simulink model "Sketch"  (R2022b)
settings: Solver=VariableStepAuto  StartTime=0.0  StopTime=10.0  RelTol=1e-3
PreLoadFcn:
  | run("Fzg_par.m")
settings Model: LastModifiedBy=timos
settings OptimizationCC: ReuseModelBlockBuffer=on
settings RTWCC: GPUComputeCapability=5.0
settings ConfigComp: CovBoundaryAbsTol=1.0e-5

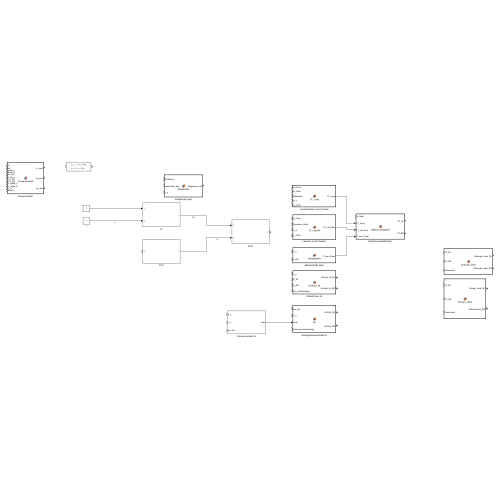
[thumbnail: Simulink's stored preview of the top-level diagram]
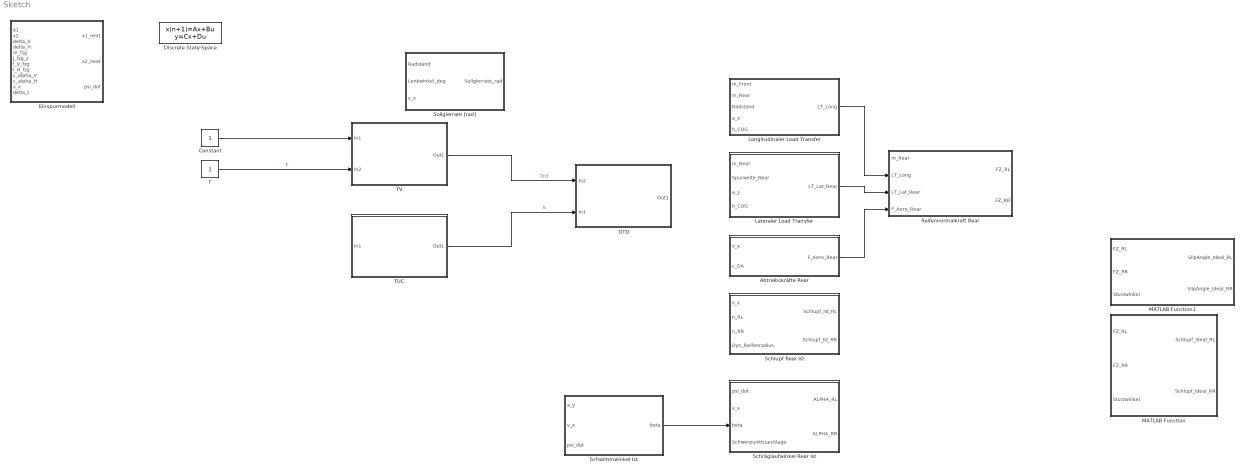
== system Sketch ==
  Abtriebskräfte Rear : MATLAB Function  TreatAsAtomicUnit=on
  Constant : Constant
  DTD : Subsystem
  Discrete State-Space : DiscreteStateSpace  SampleTime=-1
  Einspurmodell : MATLAB Function  TreatAsAtomicUnit=on
  Lateraler Load Transfer : MATLAB Function  TreatAsAtomicUnit=on
  Longitudinaler Load Transfer : MATLAB Function  TreatAsAtomicUnit=on
  MATLAB Function : MATLAB Function  TreatAsAtomicUnit=on
  MATLAB Function1 : MATLAB Function  TreatAsAtomicUnit=on
  Reifennormalkraft Rear : MATLAB Function  TreatAsAtomicUnit=on
  Schlupf Rear Ist : MATLAB Function  TreatAsAtomicUnit=on
  Schräglaufwinkel Rear Ist : MATLAB Function  TreatAsAtomicUnit=on
  Schwimmwinkel Ist : Subsystem
  Sollgierrate [rad] : MATLAB Function  TreatAsAtomicUnit=on
  TUC : Subsystem
  TV : Subsystem
  Γ : Constant
  wires:
  TUC/1(Out1) -> DTD/2(In1)  "S"
  TV/1(Out1) -> DTD/1(In2)  "Γr/l"
  Constant/1 -> TV/1(In1)
  Γ/1 -> TV/2(In2)  "Γ"
  Longitudinaler Load Transfer/1(LT_Long) -> Reifennormalkraft Rear/2(LT_Long)
  Lateraler Load Transfer/1(LT_Lat_Rear) -> Reifennormalkraft Rear/3(LT_Lat_Rear)
  Abtriebskräfte Rear/1(F_Aero_Rear) -> Reifennormalkraft Rear/4(F_Aero_Rear)
  Schwimmwinkel Ist/1(beta) -> Schräglaufwinkel Rear Ist/3(beta)

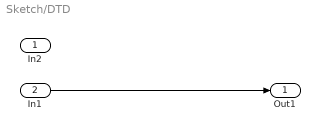
== system Sketch/DTD ==
  In2 : Inport
  In1 : Inport  Port=2
  Out1 : Outport
  wires:
  In1/1 -> Out1/1

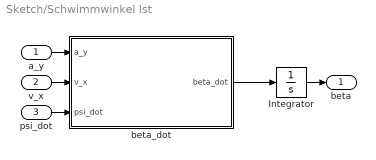
== system Sketch/Schwimmwinkel Ist ==
  a_y : Inport
  v_x : Inport  Port=2
  psi_dot : Inport  Port=3
  Integrator : Integrator
  beta_dot : MATLAB Function  TreatAsAtomicUnit=on
  beta : Outport
  wires:
  v_x/1 -> beta_dot/2(v_x)
  a_y/1 -> beta_dot/1(a_y)
  psi_dot/1 -> beta_dot/3(psi_dot)
  beta_dot/1(beta_dot) -> Integrator/1
  Integrator/1 -> beta/1

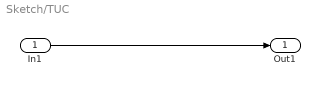
== system Sketch/TUC ==
  In1 : Inport
  Out1 : Outport
  wires:
  In1/1 -> Out1/1

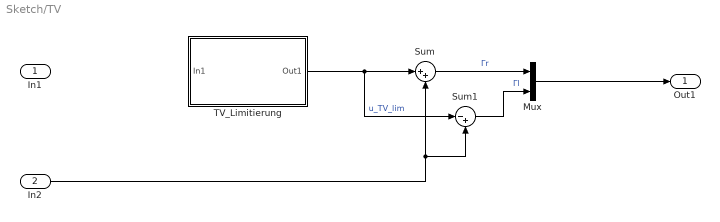
== system Sketch/TV ==
  In1 : Inport
  In2 : Inport  Port=2
  Mux : Mux  Inputs=2
  Sum : Sum  Inputs=|++
  Sum1 : Sum  Inputs=|-+
  TV_Limitierung : Subsystem
  Out1 : Outport
  wires:
  TV_Limitierung/1(Out1) -> Sum1/1, Sum/1  "u_TV_lim"
  In2/1 -> Sum1/2, Sum/2
  Sum/1 -> Mux/1  "Γr"
  Sum1/1 -> Mux/2  "Γl"
  Mux/1 -> Out1/1

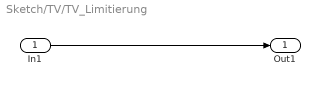
== system Sketch/TV/TV_Limitierung ==
  In1 : Inport
  Out1 : Outport
  wires:
  In1/1 -> Out1/1

== matlab function Sketch/Schräglaufwinkel Rear Ist ==
  data: psi_dot input; ALPHA_RL output; ALPHA_RR output; v_x input; beta input; Schwerpunktruecklage input
function [ALPHA_RL,ALPHA_RR] = fcn(psi_dot,v_x,beta,Schwerpunktruecklage)

    ALPHA_RL = (psi_dot*Schwerpunktruecklage/v_x) + beta;
    ALPHA_RR = ALPHA_RL;

== matlab function Sketch/Schwimmwinkel Ist/beta_dot ==
  data: a_y input; beta_dot output; v_x input; psi_dot input
function beta_dot  = Schwimmwinkel(a_y,v_x,psi_dot)

    beta_dot = (a_y/v_x) - psi_dot;

== matlab function Sketch/MATLAB Function1 ==
  data: FZ_RL input; SlipAngle_Ideal_RL output; FZ_RR input; Sturzwinkel input; SlipAngle_Ideal_RR output
function [SlipAngle_Ideal_RL,SlipAngle_Ideal_RR] = Schlupf_Ideal(FZ_RL,FZ_RR,Sturzwinkel)
% Scaling und Shape Koeffizienten
LCY   				= 0.90;
LMUY  				= 0.75;
LEY   				= 1;
LKY   				= 1;
LHY   				= 0;
LVY   				= 0;
LGAY  				= 0.75;
% Laterale Koeffizienten
PCY1				= +1.625E+000;
PDY1				= +2.554E+000;
PDY2				= -4.021E-001;
PDY3				= +5.406E+000;
PEY1				= +1.715E-001;
PEY2				= -8.339E-001;
PEY3				= -1.743E-001;
PEY4				= -6.110E+000;
PKY1				= -5.912E+001;
PKY2				= +2.567E+000;
PKY3				= +4.787E-001;
PHY1				= +0.000E+000;
PHY2				= +0.000E+000;
PHY3				= -2.152E-002;
PVY1				= +0.000E+000;
PVY2				= +0.000E+000;
PVY3				= -2.151E+000;
PVY4				= -8.772E-001;
% =======================================================================
% RL
i = 0;
Fz = FZ_RL;
GAMMA = Sturzwinkel;
FY_RL = zeros((12/0.1),3);                                                  % Vorinitialisierung
for ALPHA = 0:0.1:12
    % ====================================================================
    % Magic Formula Berechnung FX // Nur Längsschlupf
    GAMMAY = GAMMA .* LGAY;
    SHY = (PHY1 + PHY2 .* DFZ) .* LHY + PHY3 .* GAMMAY;
    ALPHAY = ALPHA + SHY;
    CY = PCY1 .* LCY;
    MUY = (PDY1 + PDY2 .* DFZ) .* (1 - PDY3 .* GAMMAY.^2) .* LMUY;
    DY = MUY .* Fz;
    EY = (PEY1 + PEY2 .* DFZ) .* (1 - (PEY3 + PEY4 .* GAMMAY) .* sign(ALPHAY)) .* LEY;
    KY = PKY1 .* FZ0 .* sin(2 * atan(Fz ./ (PKY2 .* FZ0 .* LFZO))) .* (1 - PKY3 .* abs(GAMMAY)) .* LFZO .* LKY;
    BY = KY ./ (CY .* DY);
    SVY = Fz .* ((PVY1 + PVY2 .* DFZ) .* LVY + (PVY3 + PVY4 .* DFZ) .* GAMMAY) .* LMUY;
    % ====================================================================
    % Eintragung in die Matrix
    i=i+1;
    FY_RL(i,1) = Fz;
    FY_RL(i,2) = ALPHA;
    FY_RL(i,3) = DY .* sin(CY .* atan(BY .* ALPHAY - EY .* (BY .* ALPHAY - atan(BY .* ALPHAY)))) + SVY;
end
[~, Index] = max(FY_RL(:,3));                                               % Zeilennummer des maximalen FX-Werte
SlipAngle_Ideal_RL = FY_RL(Index,2);                                        % Eintragung in die Ausgabegröße
% =======================================================================
% RR
i = 0;
Fz = FZ_RR;
GAMMA = Sturzwinkel;
FY_RR = zeros((12/0.1),3);                                                  % Vorinitialisierung
for ALPHA = 0:0.1:12
    % ====================================================================
    % Magic Formula Berechnung FX // Nur Längsschlupf
    GAMMAY = GAMMA .* LGAY;
    SHY = (PHY1 + PHY2 .* DFZ) .* LHY + PHY3 .* GAMMAY;
    ALPHAY = ALPHA + SHY;
    CY = PCY1 .* LCY;
    MUY = (PDY1 + PDY2 .* DFZ) .* (1 - PDY3 .* GAMMAY.^2) .* LMUY;
    DY = MUY .* Fz;
    EY = (PEY1 + PEY2 .* DFZ) .* (1 - (PEY3 + PEY4 .* GAMMAY) .* sign(ALPHAY)) .* LEY;
    KY = PKY1 .* FZ0 .* sin(2 * atan(Fz ./ (PKY2 .* FZ0 .* LFZO))) .* (1 - PKY3 .* abs(GAMMAY)) .* LFZO .* LKY;
    BY = KY ./ (CY .* DY);
    SVY = Fz .* ((PVY1 + PVY2 .* DFZ) .* LVY + (PVY3 + PVY4 .* DFZ) .* GAMMAY) .* LMUY;
    % ====================================================================
    % Eintragung in die Matrix
    i=i+1;
    FY_RR(i,1) = Fz;
    FY_RR(i,2) = ALPHA;
    FY_RR(i,3) = DY .* sin(CY .* atan(BY .* ALPHAY - EY .* (BY .* ALPHAY - atan(BY .* ALPHAY)))) + SVY;
end
[~, Index] = max(FY_RR(:,3));                                               % Zeilennummer des maximalen FX-Werte
SlipAngle_Ideal_RR = FY_RR(Index,2);                                        % Eintragung in die Ausgabegröße

== matlab function Sketch/MATLAB Function ==
  data: FZ_RL input; Schlupf_Ideal_RL output; FZ_RR input; Sturzwinkel input; Schlupf_Ideal_RR output
function [Schlupf_Ideal_RL,Schlupf_Ideal_RR] = Schlupf_Ideal(FZ_RL,FZ_RR,Sturzwinkel)
% =======================================================================
% Magic Formula Parameter
% Scaling und Shape Koeffizienten
LCX   				= 1;
LMUX  				= 0.75;
LEX   				= 1;
LKX   				= 1;
LHX   				= 1;
LVX   				= 1;
LGAX  				= 1;
% Longitudinal Koeffizienten
PCX1  				= +1.786E+000;
PDX1  				= +2.688E+000;
PDX2  				= -2.720E-001;
PDX3  				= +1.370E+001;
PEX1  				= +8.710E-001;
PEX2  				= -3.800E-002;
PEX3  				= +0.000E+000;
PEX4  				= +7.100E-002;
PKX1  				= +8.125E+001;
PKX2  				= -2.025E+001;
PKX3  				= +5.000E-001;
PHX1  				= +0.000E+000;
PHX2  				= +0.000E+000;
PVX1  				= +0.000E+000;
PVX2  				= +0.000E+000;
% =======================================================================
% RL
i = 0;
Fz = FZ_RL;
GAMMA = Sturzwinkel;
FX_RL = zeros((0.3/0.01),3);                                                % Vorinitialisierung
for KAPPA = 0:0.01:0.3
    % ====================================================================
    % Magic Formula Berechnung FX // Nur Längsschlupf
    GAMMAX = GAMMA .* LGAX;
    SHX = (PHX1 + PHX2 .* DFZ) .* LHX;
    KAPPAX = KAPPA + SHX;
    CX = PCX1 .* LCX;
    MUX = (PDX1 + PDX2 .* DFZ) .* (1 - PDX3 .* GAMMAX.^2) .* LMUX;
    DX = MUX .* Fz;
    EX = (PEX1 + PEX2 .* DFZ + PEX3 .* DFZ.^2) .* (1 - PEX4 .* sign(KAPPAX)) .* LEX;
    KX = Fz .* (PKX1 + PKX2 .* DFZ) .* exp(PKX3 .* DFZ) .* LKX;
    BX = KX ./ (CX .* DX);
    SVX = Fz .* (PVX1 + PVX2 .* DFZ) .* LVX .* LMUX;
    % ====================================================================
    % Eintragung in die Matrix
    i=i+1;
    FX_RL(i,1) = Fz;
    FX_RL(i,2) = KAPPA;
    FX_RL(i,3) = DX .* sin(CX .* atan(BX .* KAPPAX - EX .* (BX .* KAPPAX - atan(BX .* KAPPAX)))) + SVX;
end
[~, Index] = max(FX_RL(:,3));                                               % Zeilennummer des maximalen FX-Werte
Schlupf_Ideal_RL = FX_RL(Index,:);                                          % Eintragung in die Ausgabegröße
% =======================================================================
% RR
i = 0;
Fz = FZ_RR;
GAMMA = Sturzwinkel;
FX_RR = zeros((0.3/0.01),3);                                                % Vorinitialisierung
for KAPPA = 0:0.01:0.3
    % ====================================================================
    % Magic Formula Berechnung FX // Nur Längsschlupf
    GAMMAX = GAMMA .* LGAX;
    SHX = (PHX1 + PHX2 .* DFZ) .* LHX;
    KAPPAX = KAPPA + SHX;
    CX = PCX1 .* LCX;
    MUX = (PDX1 + PDX2 .* DFZ) .* (1 - PDX3 .* GAMMAX.^2) .* LMUX;
    DX = MUX .* Fz;
    EX = (PEX1 + PEX2 .* DFZ + PEX3 .* DFZ.^2) .* (1 - PEX4 .* sign(KAPPAX)) .* LEX;
    KX = Fz .* (PKX1 + PKX2 .* DFZ) .* exp(PKX3 .* DFZ) .* LKX;
    BX = KX ./ (CX .* DX);
    SVX = Fz .* (PVX1 + PVX2 .* DFZ) .* LVX .* LMUX;
    % ====================================================================
    % Eintragung in die Matrix
    i=i+1;
    FX_RR(i,1) = Fz;
    FX_RR(i,2) = KAPPA;
    FX_RR(i,3) = DX .* sin(CX .* atan(BX .* KAPPAX - EX .* (BX .* KAPPAX - atan(BX .* KAPPAX)))) + SVX;
end
[~, Index] = max(FX_RR(:,3));                                               % Zeilennummer des maximalen FX-Werte
Schlupf_Ideal_RR = FX_RR(Index,:);                                          % Eintragung in die Ausgabegröße

== matlab function Sketch/Schlupf Rear Ist ==
  data: v_x input; Schlupf_Ist_RL output; n_RL input; n_RR input; Dyn_Reifenradius input; Schlupf_Ist_RR output
function [Schlupf_Ist_RL,Schlupf_Ist_RR]   = Schlupf_Ist(v_x,n_RL,n_RR,Dyn_Reifenradius)

    n_x = v_x / (pi*Dyn_Reifenradius);
    Schlupf_Ist_RL = (n_RL-n_x)/n_x;
    Schlupf_Ist_RR = (n_RR-n_x)/n_x;

== matlab function Sketch/Sollgierrate [rad] ==
  data: Radstand input; Sollgierrate_rad output; Lenkwinkel_deg input; v_x input
function Sollgierrate_rad = Sollgierrate(Radstand,Lenkwinkel_deg,v_x)
    
    Sollgierrate_rad = deg2rad(Lenkwinkel_deg) * v_x / Radstand;

== matlab function Sketch/Lateraler Load Transfer ==
  data: LT_Lat_Rear output; m_Rear input; Spurweite_Rear input; a_y input; h_COG input
function LT_Lat_Rear  = LT_Lateral(m_Rear,Spurweite_Rear,a_y,h_COG)

    LT_Lat_Rear = m_Rear*a_y*h_COG / Spurweite_Rear;

== matlab function Sketch/Longitudinaler Load Transfer ==
  data: m_Front input; LT_Long output; m_Rear input; Radstand input; a_x input; h_COG input
function LT_Long  = LT_Long(m_Front,m_Rear,Radstand,a_x,h_COG)

    LT_Long = (m_Front+m_Rear)*a_x*h_COG / Radstand;

== matlab function Sketch/Einspurmodell ==
  data: x1 input; x1_next output; x2 input; delta_V input; delta_H input; m_fzg input; J_fzg_z input; l_V_fzg input; l_H_fzg input; c_alpha_V input; c_alpha_H input; v_x input; delta_t input; x2_next output; psi_dot output
function [x1_next, x2_next, psi_dot] = Einspurmodell(x1, x2, delta_V, delta_H, m_fzg, J_fzg_z, l_V_fzg, l_H_fzg, c_alpha_V, c_alpha_H, v_x, delta_t)
%#codegen

% Systemmatrizen bei aktuellem v_x und delta_V berechnen
A = [-(c_alpha_V*l_V_fzg^2+c_alpha_H*l_H_fzg^2)/(J_fzg_z*v_x), (c_alpha_H*l_H_fzg-c_alpha_V*l_V_fzg)/J_fzg_z;
     (c_alpha_H*l_H_fzg-c_alpha_V*l_V_fzg-m_fzg*v_x^2)/(m_fzg*v_x^2), -(c_alpha_V+c_alpha_H)/(m_fzg*v_x)];

B = [(c_alpha_V*l_V_fzg)/J_fzg_z, -(c_alpha_H*l_H_fzg)/J_fzg_z;
      c_alpha_V/(m_fzg*v_x),        c_alpha_H/(m_fzg*v_x)];

C = [1 0];

% Zustandsupdate mit Euler-Diskretisierung
x1_next = x1 + delta_t*(A(1,1)*x1 + A(1,2)*x2 + B(1,1)*delta_V + B(1,2)*delta_H);
x2_next = x2 + delta_t*(A(2,1)*x1 + A(2,2)*x2 + B(2,1)*delta_V + B(2,2)*delta_H);

% Ausgang
psi_dot = C(1)*x1 + C(2)*x2;
end

== matlab function Sketch/Reifennormalkraft Rear ==
  data: m_Rear input; FZ_RL output; LT_Long input; LT_Lat_Rear input; F_Aero_Rear input; FZ_RR output
function [FZ_RL,FZ_RR] = Reifennormalkraft(m_Rear,LT_Long,LT_Lat_Rear,F_Aero_Rear)

    FZ_RL = (m_Rear*9.81) + LT_Long/4 + LT_Lat_Rear/2 + F_Aero_Rear/2;
    FZ_RR = (m_Rear*9.81) + LT_Long/4 - LT_Lat_Rear/2 + F_Aero_Rear/2;

== matlab function Sketch/Abtriebskräfte Rear ==
  data: v_x input; F_Aero_Rear output; c_DA input
function F_Aero_Rear   = Abriebskraft(v_x,c_DA)

    F_Aero_Rear = 0.5 * 1.225 * c_DA * v_x * v_x;
